simulink model "PIntkVUs_DD"  (R2016b)
settings: configuration reference "CodeGenConfigSet" (kept outside this file)
values from neighbouring files (symbols this model uses):
  Air_facPT1T1PIntkVUs_C = Calibration.Parameter    [init_PIntkVUs_DD.m]
  Air_pMaxDiffLimPlsPIntkVUs_C = Calibration.Parameter    [init_PIntkVUs_DD.m]
  Air_pMinDiffLimPlsPIntkVUs_C = Calibration.Parameter    [init_PIntkVUs_DD.m]
  Air_pPhysRngPIntkVUsMax_C = Calibration.Parameter    [init_PIntkVUs_DD.m]
  Air_pPhysRngPIntkVUsMin_C = Calibration.Parameter    [init_PIntkVUs_DD.m]
  Air_pTransfPIntkVUs_CUR = Calibration.Parameter    [init_PIntkVUs_DD.m]
  Air_pTransfPIntkVUs_CURX = Calibration.Parameter    [init_PIntkVUs_DD.m]
  Air_tiPhysRngHiIntkVUsDefDeb_C = Calibration.Parameter    [init_PIntkVUs_DD.m]
  Air_tiPhysRngHiIntkVUsOKDeb_C = Calibration.Parameter    [init_PIntkVUs_DD.m]
  Air_tiPhysRngLoIntkVUsDefDeb_C = Calibration.Parameter    [init_PIntkVUs_DD.m]
  Air_tiPhysRngLoIntkVUsOKDeb_C = Calibration.Parameter    [init_PIntkVUs_DD.m]
  Air_tiPIntkVUsMaxDefDeb_C = Calibration.Parameter    [init_PIntkVUs_DD.m]
  Air_tiPIntkVUsMaxOKDeb_C = Calibration.Parameter    [init_PIntkVUs_DD.m]
  Air_tiPIntkVUsMinDefDeb_C = Calibration.Parameter    [init_PIntkVUs_DD.m]
  Air_tiPIntkVUsMinOKDeb_C = Calibration.Parameter    [init_PIntkVUs_DD.m]
  Air_tiPlsMaxIntkVUsDefDeb_C = Calibration.Parameter    [init_PIntkVUs_DD.m]
  Air_tiPlsMaxIntkVUsOKDeb_C = Calibration.Parameter    [init_PIntkVUs_DD.m]
  Air_tiPlsMinIntkVUsDefDeb_C = Calibration.Parameter    [init_PIntkVUs_DD.m]
  Air_tiPlsMinIntkVUsOKDeb_C = Calibration.Parameter    [init_PIntkVUs_DD.m]
  Air_uSRCPIntkVUsMax_C = Calibration.Parameter    [init_PIntkVUs_DD.m]
  Air_uSRCPIntkVUsMin_C = Calibration.Parameter    [init_PIntkVUs_DD.m]
undefined symbols (not defined in the file or in its folder): EpmSynState_conv, PIntkVUs_DD_DT
libraries: CXLib x19
settings Model: Creator=GaberXu  LastModifiedBy=wangrui
settings ConfigSetRef: SourceLocation=Base Workspace

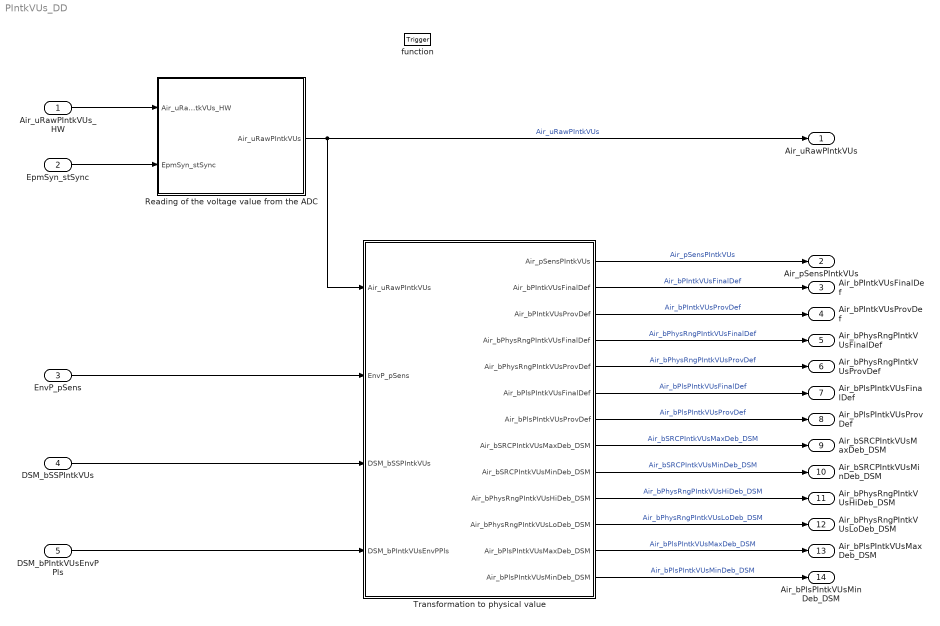
== system PIntkVUs_DD ==
  Air_uRawPIntkVUs_HW : Inport  Tag=mv  Description=Raw ADC value of air pressure upstream of the intake valve  OutMin=0  OutMax=5000  OutDataTypeStr=Ad_mv
  EpmSyn_stSync : Inport  Description=state of synchronization  Port=2  OutDataTypeStr=Enum:EpmSynState_conv
  EnvP_pSens : Inport  Tag=kPa  Description=Raw physical value  Port=3  OutMin=0  OutMax=1200  OutDataTypeStr=AirPressure_kPa
  DSM_bSSPIntkVUs : Inport  Description=State of FId_SSPIntkVUs  Port=4  OutMin=0  OutMax=1  OutDataTypeStr=boolean
  DSM_bPIntkVUsEnvPPls : Inport  Description=State of FId_PIntkVUsEnvPPls  Port=5  OutMin=0  OutMax=1  OutDataTypeStr=boolean
  function : TriggerPort  TriggerType=function-call  VariantControl=Variant
  Reading of the voltage value from the ADC : Subsystem
  Transformation to physical value : Subsystem
  Air_uRawPIntkVUs : Outport  Tag=mv  Description=Averaging raw ADC value of air pressure upstream of the intake valve  OutMin=0  OutMax=5000  OutDataTypeStr=Ad_mv
  Air_pSensPIntkVUs : Outport  Tag=kPa  Description=Sensed manifold absolute pressure  Port=2  OutMin=0  OutMax=1200  OutDataTypeStr=AirPressure_kPa
  Air_bPIntkVUsFinalDef : Outport  Description=Final defect of the raw air pressure upstream of the intake valve  Port=3  OutMin=0  OutMax=1  OutDataTypeStr=boolean
  Air_bPIntkVUsProvDef : Outport  Description=Provisional defect of the raw air pressure upstream of the intake valve  Port=4  OutMin=0  OutMax=1  OutDataTypeStr=boolean
  Air_bPhysRngPIntkVUsFinalDef : Outport  Description=Final defect of the physical air pressure upstream of the intake valve  Port=5  OutMin=0  OutMax=1  OutDataTypeStr=boolean
  Air_bPhysRngPIntkVUsProvDef : Outport  Description=Provisional defect of the physical air pressure upstream of the intake valve  Port=6  OutMin=0  OutMax=1  OutDataTypeStr=boolean
  Air_bPlsPIntkVUsFinalDef : Outport  Description=Final defect which the air pressure upstream of the intake valve is not plausible  Port=7  OutMin=0  OutMax=1  OutDataTypeStr=boolean
  Air_bPlsPIntkVUsProvDef : Outport  Description=Provisional defect which the air pressure upstream of the intake valve is not plausible  Port=8  OutMin=0  OutMax=1  OutDataTypeStr=boolean
  Air_bSRCPIntkVUsMaxDeb_DSM : Outport  Description=DSM defect which the raw air pressure upstream of the intake valve is exceeding the maximum in SRC  Port=9  OutMin=0  OutMax=1  OutDataTypeStr=boolean
  Air_bSRCPIntkVUsMinDeb_DSM : Outport  Description=DSM defect which the raw air pressure upstream of the intake valve is exceeding the minimum in SRC  Port=10  OutMin=0  OutMax=1  OutDataTypeStr=boolean
  Air_bPhysRngPIntkVUsHiDeb_DSM : Outport  Description="DSM defect which the physical  air pressure upstream of the intake valve is exceeding the highest value in SRC"  Port=11  OutMin=0  OutMax=1  OutDataTypeStr=boolean
  Air_bPhysRngPIntkVUsLoDeb_DSM : Outport  Description="DSM defect which the physical  air pressure upstream of the intake valve is exceeding the lowest value in SRC"  Port=12  OutMin=0  OutMax=1  OutDataTypeStr=boolean
  Air_bPlsPIntkVUsMaxDeb_DSM : Outport  Description=DSM defect which the air pressure upstream of the intake valve is exceeding the maximum in plausibility check  Port=13  OutMin=0  OutMax=1  OutDataTypeStr=boolean
  Air_bPlsPIntkVUsMinDeb_DSM : Outport  Description=DSM defect which the air pressure upstream of the intake valve is exceeding the minimum in plausibility check  Port=14  OutMin=0  OutMax=1  OutDataTypeStr=boolean
  wires:
  Reading of the voltage value from the ADC/1(Air_uRawPIntkVUs) -> Air_uRawPIntkVUs/1, Transformation to physical value/1(Air_uRawPIntkVUs)  "Air_uRawPIntkVUs"
  Transformation to physical value/1(Air_pSensPIntkVUs) -> Air_pSensPIntkVUs/1  "Air_pSensPIntkVUs"
  Transformation to physical value/2(Air_bPIntkVUsFinalDef) -> Air_bPIntkVUsFinalDef/1  "Air_bPIntkVUsFinalDef"
  Transformation to physical value/3(Air_bPIntkVUsProvDef) -> Air_bPIntkVUsProvDef/1  "Air_bPIntkVUsProvDef"
  Transformation to physical value/4(Air_bPhysRngPIntkVUsFinalDef) -> Air_bPhysRngPIntkVUsFinalDef/1  "Air_bPhysRngPIntkVUsFinalDef"
  Transformation to physical value/5(Air_bPhysRngPIntkVUsProvDef) -> Air_bPhysRngPIntkVUsProvDef/1  "Air_bPhysRngPIntkVUsProvDef"
  Transformation to physical value/6(Air_bPlsPIntkVUsFinalDef) -> Air_bPlsPIntkVUsFinalDef/1  "Air_bPlsPIntkVUsFinalDef"
  Transformation to physical value/7(Air_bPlsPIntkVUsProvDef) -> Air_bPlsPIntkVUsProvDef/1  "Air_bPlsPIntkVUsProvDef"
  Transformation to physical value/8(Air_bSRCPIntkVUsMaxDeb_DSM) -> Air_bSRCPIntkVUsMaxDeb_DSM/1  "Air_bSRCPIntkVUsMaxDeb_DSM"
  Transformation to physical value/9(Air_bSRCPIntkVUsMinDeb_DSM) -> Air_bSRCPIntkVUsMinDeb_DSM/1  "Air_bSRCPIntkVUsMinDeb_DSM"
  Transformation to physical value/10(Air_bPhysRngPIntkVUsHiDeb_DSM) -> Air_bPhysRngPIntkVUsHiDeb_DSM/1  "Air_bPhysRngPIntkVUsHiDeb_DSM"
  Transformation to physical value/11(Air_bPhysRngPIntkVUsLoDeb_DSM) -> Air_bPhysRngPIntkVUsLoDeb_DSM/1  "Air_bPhysRngPIntkVUsLoDeb_DSM"
  Transformation to physical value/12(Air_bPlsPIntkVUsMaxDeb_DSM) -> Air_bPlsPIntkVUsMaxDeb_DSM/1  "Air_bPlsPIntkVUsMaxDeb_DSM"
  Transformation to physical value/13(Air_bPlsPIntkVUsMinDeb_DSM) -> Air_bPlsPIntkVUsMinDeb_DSM/1  "Air_bPlsPIntkVUsMinDeb_DSM"
  EpmSyn_stSync/1 -> Reading of the voltage value from the ADC/2(EpmSyn_stSync)
  Air_uRawPIntkVUs_HW/1 -> Reading of the voltage value from the ADC/1(Air_uRawPIntkVUs_HW)
  EnvP_pSens/1 -> Transformation to physical value/2(EnvP_pSens)
  DSM_bSSPIntkVUs/1 -> Transformation to physical value/3(DSM_bSSPIntkVUs)
  DSM_bPIntkVUsEnvPPls/1 -> Transformation to physical value/4(DSM_bPIntkVUsEnvPPls)

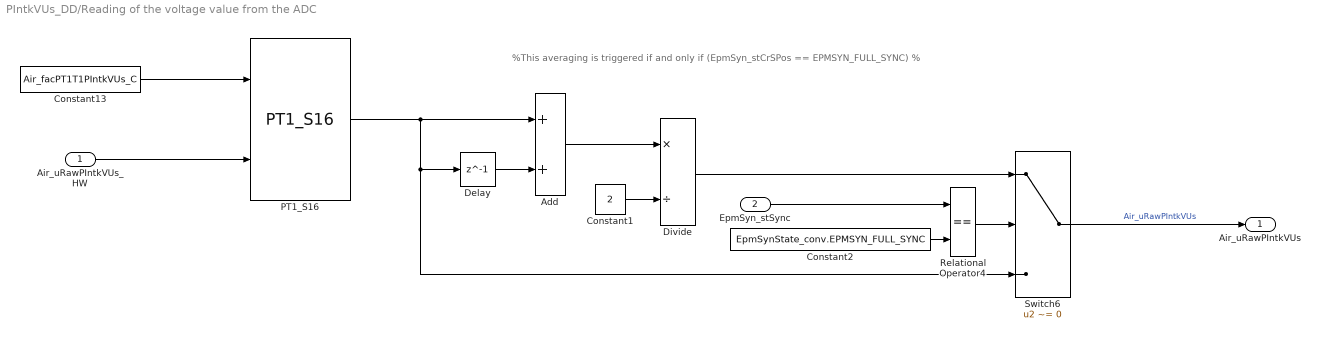
== system PIntkVUs_DD/Reading of the voltage value from the ADC ==
  note: %This averaging is triggered if and only if (EpmSyn_stCrSPos == EPMSYN_FULL_SYNC) %
  Air_uRawPIntkVUs_HW : Inport
  EpmSyn_stSync : Inport  Port=2
  Add : Sum  SaturateOnIntegerOverflow=on  InputSameDT=on
  Constant1 : Constant  Value=2  OutDataTypeStr=uint16
  Constant13 : Constant  Value=Air_facPT1T1PIntkVUs_C
  Constant2 : Constant  Value=EpmSynState_conv.EPMSYN_FULL_SYNC
  Delay : Delay  DelayLength=1  InitialCondition=0
  Divide : Product  Inputs=*/  OutDataTypeStr=Ad_mv  SaturateOnIntegerOverflow=on
  PT1_S16 : CXLib/PT1_S16  offset=0
  Relational Operator4 : RelationalOperator  Operator===  OutDataTypeStr=boolean  RndMeth=Nearest  InputSameDT=on
  Switch6 : Switch  Criteria=u2 ~= 0  InputSameDT=on
  Air_uRawPIntkVUs : Outport
  wires:
  Air_uRawPIntkVUs_HW/1 -> PT1_S16/2
  Constant1/1 -> Divide/2
  Relational Operator4/1 -> Switch6/2
  Divide/1 -> Switch6/1
  Delay/1 -> Add/2
  Switch6/1 -> Air_uRawPIntkVUs/1  "Air_uRawPIntkVUs"
  EpmSyn_stSync/1 -> Relational Operator4/1
  Add/1 -> Divide/1
  Constant2/1 -> Relational Operator4/2
  Constant13/1 -> PT1_S16/1
  PT1_S16/1 -> Switch6/3, Delay/1, Add/1

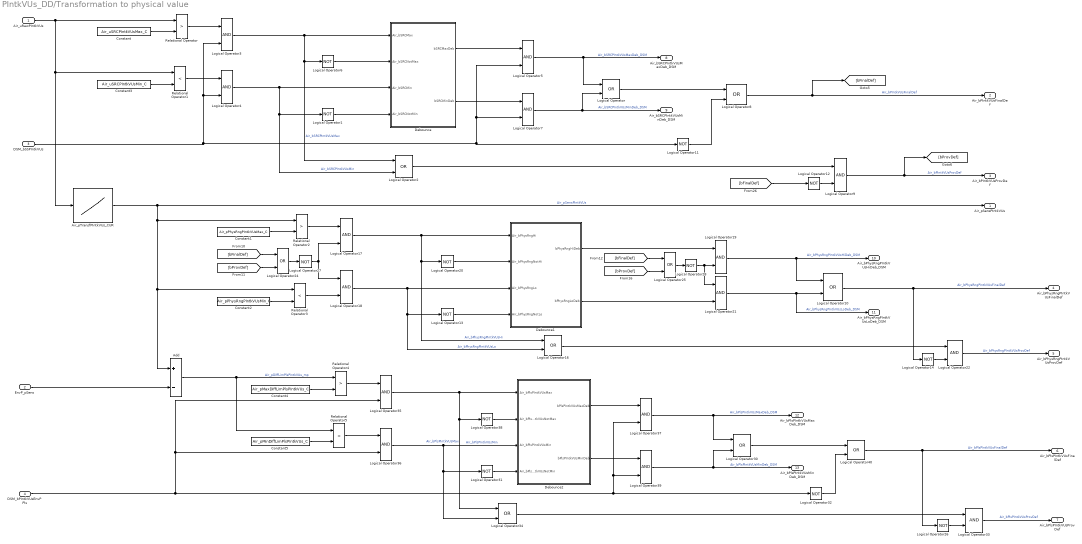
== system PIntkVUs_DD/Transformation to physical value ==
  Air_uRawPIntkVUs : Inport
  EnvP_pSens : Inport  Port=2
  DSM_bSSPIntkVUs : Inport  Port=3
  DSM_bPIntkVUsEnvPPls : Inport  Port=4
  Add : Sum  Inputs=+-  SaturateOnIntegerOverflow=on  InputSameDT=on
  Air_pTransfPIntkVUs_CUR : Lookup_n-D  NumberOfTableDimensions=1  BreakpointsForDimension1=Air_pTransfPIntkVUs_CURX  IndexSearchMethod=Linear search  BeginIndexSearchUsingPreviousIndexResult=on  UseOneInputPortForAllInputData=on  Table=Air_pTransfPIntkVUs_CUR  ExtrapMethod=Clip  UseLastTableValue=on  InternalRulePriority=Speed  OutDataTypeStr=Inherit: Inherit via back propagation  SaturateOnIntegerOverflow=on
  Constant : Constant  Value=Air_uSRCPIntkVUsMax_C
  Constant1 : Constant  Value=Air_pPhysRngPIntkVUsMax_C
  Constant2 : Constant  Value=Air_pPhysRngPIntkVUsMin_C
  Constant3 : Constant  Value=Air_uSRCPIntkVUsMin_C
  Constant4 : Constant  Value=Air_pMaxDiffLimPlsPIntkVUs_C
  Constant5 : Constant  Value=Air_pMinDiffLimPlsPIntkVUs_C
  Debounce : Subsystem
  Debounce1 : Subsystem
  Debounce2 : Subsystem
  Logical Operator{,2,8,10,16,30,34,40} (8 alike) : Logic  Operator=OR  AllPortsSameDT=off  OutDataTypeStr=boolean
  Logical Operator{1,6,11..14,20,26..28,31..32,38} (13 alike) : Logic  Operator=NOT  AllPortsSameDT=off  OutDataTypeStr=boolean
  Logical Operator{3..5,7,9,17..19,21..22,33,35..37,39} (15 alike) : Logic  AllPortsSameDT=off  OutDataTypeStr=boolean
  Logical Operator24 : Logic  RequirementInfo={} %GIDa_41b44013_9ec1_49ef_a77d_a735944319c0  Operator=OR  OutDataTypeStr=boolean
  Logical Operator25 : Logic  RequirementInfo={} %GIDa_cee60f6c_ce8d_407f_bb4c_290855d67459  Operator=OR  OutDataTypeStr=boolean
  Relational Operator : RelationalOperator  Operator=>  OutDataTypeStr=boolean  RndMeth=Nearest  InputSameDT=on
  Relational Operator1 : RelationalOperator  Operator=<  OutDataTypeStr=boolean  RndMeth=Nearest  InputSameDT=on
  Relational Operator2 : RelationalOperator  Operator=>  OutDataTypeStr=boolean  RndMeth=Nearest  InputSameDT=on
  Relational Operator3 : RelationalOperator  Operator=<  OutDataTypeStr=boolean  RndMeth=Nearest  InputSameDT=on
  Relational Operator4 : RelationalOperator  Operator=>  OutDataTypeStr=boolean  RndMeth=Nearest  InputSameDT=on
  Relational Operator5 : RelationalOperator  Operator=<  OutDataTypeStr=boolean  RndMeth=Nearest  InputSameDT=on
  Air_pSensPIntkVUs : Outport
  Air_bPIntkVUsFinalDef : Outport  Port=2
  Air_bPIntkVUsProvDef : Outport  Port=3
  Air_bPhysRngPIntkVUsFinalDef : Outport  Port=4
  Air_bPhysRngPIntkVUsProvDef : Outport  Port=5
  Air_bPlsPIntkVUsFinalDef : Outport  Port=6
  Air_bPlsPIntkVUsProvDef : Outport  Port=7
  Air_bSRCPIntkVUsMaxDeb_DSM : Outport  Port=8
  Air_bSRCPIntkVUsMinDeb_DSM : Outport  Port=9
  Air_bPhysRngPIntkVUsHiDeb_DSM : Outport  Port=10
  Air_bPhysRngPIntkVUsLoDeb_DSM : Outport  Port=11
  Air_bPlsPIntkVUsMaxDeb_DSM : Outport  Port=12
  Air_bPlsPIntkVUsMinDeb_DSM : Outport  Port=13
  wires:
  Logical Operator33/1 -> Air_bPlsPIntkVUsProvDef/1  "Air_bPlsPIntkVUsProvDef"
  Logical Operator34/1 -> Logical Operator33/1
  Logical Operator26/1 -> Logical Operator33/2
  Logical Operator22/1 -> Air_bPhysRngPIntkVUsProvDef/1  "Air_bPhysRngPIntkVUsProvDef"
  Logical Operator14/1 -> Logical Operator22/2
  Debounce2/1(bPlsPIntkVUsMaxDeb) -> Logical Operator37/1
  Logical Operator31/1 -> Debounce2/4(Air_bPlsPIntkVUsNotMin)
  Logical Operator38/1 -> Debounce2/2(Air_bPlsPIntkVUsNotMax)
  Add/1 -> Relational Operator4/1, Relational Operator5/1  "Air_pDiffLimPlsPIntkVUs_mp"
  Logical Operator32/1 -> Logical Operator40/2
  Logical Operator40/1 -> Air_bPlsPIntkVUsFinalDef/1, Logical Operator26/1  "Air_bPlsPIntkVUsFinalDef"
  DSM_bPIntkVUsEnvPPls/1 -> Logical Operator32/1, Logical Operator37/2, Logical Operator39/2, Logical Operator35/2, Logical Operator36/2
  Logical Operator30/1 -> Logical Operator40/1
  Debounce2/2(bPlsPIntkVUsMinDeb) -> Logical Operator39/1
  Relational Operator5/1 -> Logical Operator36/1
  Relational Operator4/1 -> Logical Operator35/1
  Logical Operator39/1 -> Logical Operator30/2, Air_bPlsPIntkVUsMinDeb_DSM/1  "Air_bPlsPIntkVUsMinDeb_DSM"
  Logical Operator37/1 -> Air_bPlsPIntkVUsMaxDeb_DSM/1, Logical Operator30/1  "Air_bPlsPIntkVUsMaxDeb_DSM"
  Logical Operator36/1 -> Debounce2/3(Air_bPlsPIntkVUsMin), Logical Operator34/2, Logical Operator31/1  "Air_bPlsPIntkVUsMin"
  Constant5/1 -> Relational Operator5/2
  Logical Operator35/1 -> Debounce2/1(Air_bPlsPIntkVUsMax), Logical Operator34/1, Logical Operator38/1  "Air_bPlsPIntkVUsMax"
  Constant4/1 -> Relational Operator4/2
  EnvP_pSens/1 -> Add/2
  Logical Operator28/1 -> Logical Operator19/2, Logical Operator21/1
  Logical Operator27/1 -> Logical Operator17/2, Logical Operator18/1
  Debounce1/2(bPhysRngLoDeb) -> Logical Operator21/2
  [bProvDef] -> Logical Operator25/2
  [bFinalDef] -> Logical Operator25/1
  [bProvDef] -> Logical Operator24/2
  [bFinalDef] -> Logical Operator24/1
  Relational Operator3/1 -> Logical Operator18/2
  Debounce1/1(bPhysRngHiDeb) -> Logical Operator19/1
  Logical Operator13/1 -> Debounce1/4(Air_bPhysRngNotLo)
  Logical Operator20/1 -> Debounce1/2(Air_bPhysRngNotHi)
  Logical Operator10/1 -> Logical Operator14/1, Air_bPhysRngPIntkVUsFinalDef/1  "Air_bPhysRngPIntkVUsFinalDef"
  Logical Operator16/1 -> Logical Operator22/1
  Logical Operator25/1 -> Logical Operator28/1
  Logical Operator24/1 -> Logical Operator27/1
  Relational Operator2/1 -> Logical Operator17/1
  Logical Operator21/1 -> Air_bPhysRngPIntkVUsLoDeb_DSM/1, Logical Operator10/2  "Air_bPhysRngPIntkVUsLoDeb_DSM"
  Logical Operator19/1 -> Air_bPhysRngPIntkVUsHiDeb_DSM/1, Logical Operator10/1  "Air_bPhysRngPIntkVUsHiDeb_DSM"
  Logical Operator18/1 -> Debounce1/3(Air_bPhysRngLo), Logical Operator16/2, Logical Operator13/1  "Air_bPhysRngPIntkVUsLo"
  Constant2/1 -> Relational Operator3/2
  Logical Operator17/1 -> Debounce1/1(Air_bPhysRngHi), Logical Operator20/1, Logical Operator16/1  "Air_bPhysRngPIntkVUsHi"
  Constant1/1 -> Relational Operator2/2
  Air_pTransfPIntkVUs_CUR/1 -> Relational Operator2/1, Relational Operator3/1, Add/1, Air_pSensPIntkVUs/1  "Air_pSensPIntkVUs"
  Debounce/2(bSRCMinDeb) -> Logical Operator7/1
  Debounce/1(bSRCMaxDeb) -> Logical Operator5/1
  Logical Operator1/1 -> Debounce/4(Air_bSRCNotMin)
  Logical Operator6/1 -> Debounce/2(Air_bSRCNotMax)
  Air_uRawPIntkVUs/1 -> Relational Operator/1, Relational Operator1/1, Air_pTransfPIntkVUs_CUR/1
  Logical Operator12/1 -> Logical Operator9/2
  Logical Operator11/1 -> Logical Operator8/2
  Logical Operator9/1 -> [bProvDef], Air_bPIntkVUsProvDef/1  "Air_bPIntkVUsProvDef"
  Logical Operator8/1 -> Air_bPIntkVUsFinalDef/1, [bFinalDef]  "Air_bPIntkVUsFinalDef"
  [bFinalDef] -> Logical Operator12/1
  Logical Operator2/1 -> Logical Operator9/1
  DSM_bSSPIntkVUs/1 -> Logical Operator5/2, Logical Operator7/2, Logical Operator11/1, Logical Operator3/2, Logical Operator4/2
  Logical Operator/1 -> Logical Operator8/1
  Relational Operator1/1 -> Logical Operator4/1
  Relational Operator/1 -> Logical Operator3/1
  Logical Operator7/1 -> Air_bSRCPIntkVUsMinDeb_DSM/1, Logical Operator/2  "Air_bSRCPIntkVUsMinDeb_DSM"
  Logical Operator5/1 -> Air_bSRCPIntkVUsMaxDeb_DSM/1, Logical Operator/1  "Air_bSRCPIntkVUsMaxDeb_DSM"
  Logical Operator4/1 -> Debounce/3(Air_bSRCMin), Logical Operator1/1, Logical Operator2/2  "Air_bSRCPIntkVUsMin"
  Constant3/1 -> Relational Operator1/2
  Logical Operator3/1 -> Debounce/1(Air_bSRCMax), Logical Operator6/1, Logical Operator2/1  "Air_bSRCPIntkVUsMax"
  Constant/1 -> Relational Operator/2

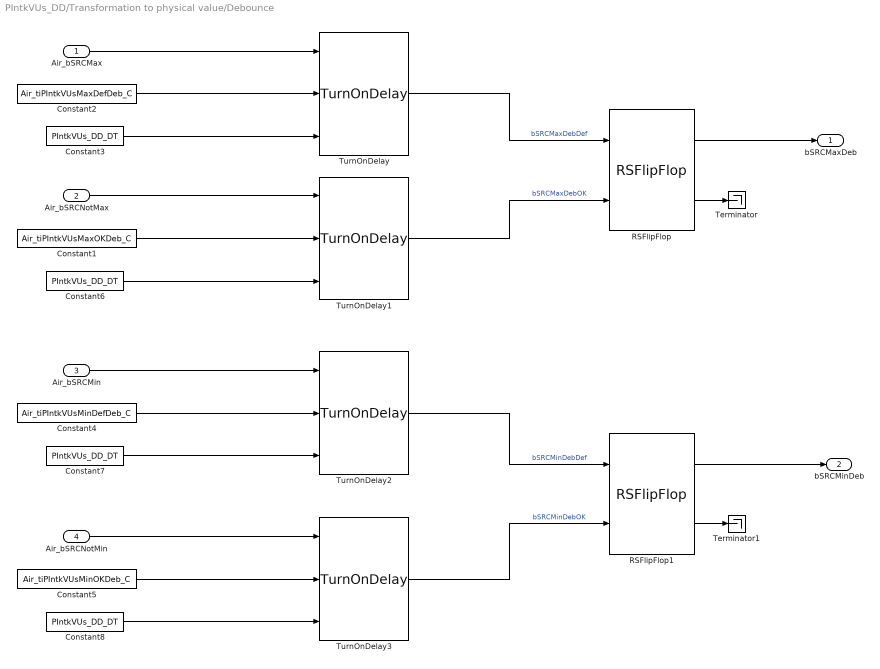
== system PIntkVUs_DD/Transformation to physical value/Debounce ==
  Air_bSRCMax : Inport
  Air_bSRCNotMax : Inport  Port=2
  Air_bSRCMin : Inport  Port=3
  Air_bSRCNotMin : Inport  Port=4
  Constant1 : Constant  Value=Air_tiPIntkVUsMaxOKDeb_C
  Constant2 : Constant  Value=Air_tiPIntkVUsMaxDefDeb_C
  Constant{3,6..8} (4 alike) : Constant  Value=PIntkVUs_DD_DT
  Constant4 : Constant  Value=Air_tiPIntkVUsMinDefDeb_C
  Constant5 : Constant  Value=Air_tiPIntkVUsMinOKDeb_C
  RSFlipFlop : CXLib/RSFlipFlop
  RSFlipFlop1 : CXLib/RSFlipFlop
  Terminator : Terminator
  Terminator1 : Terminator
  TurnOnDelay{,1..3} (4 alike) : CXLib/TurnOnDelay
  bSRCMaxDeb : Outport
  bSRCMinDeb : Outport  Port=2
  wires:
  Constant8/1 -> TurnOnDelay3/3
  Constant7/1 -> TurnOnDelay2/3
  Constant6/1 -> TurnOnDelay1/3
  Constant3/1 -> TurnOnDelay/3
  Air_bSRCMax/1 -> TurnOnDelay/1
  RSFlipFlop1/2 -> Terminator1/1
  RSFlipFlop/2 -> Terminator/1
  Constant5/1 -> TurnOnDelay3/2
  TurnOnDelay3/1 -> RSFlipFlop1/2  "bSRCMinDebOK"
  Air_bSRCNotMin/1 -> TurnOnDelay3/1
  TurnOnDelay2/1 -> RSFlipFlop1/1  "bSRCMinDebDef"
  Air_bSRCMin/1 -> TurnOnDelay2/1
  Air_bSRCNotMax/1 -> TurnOnDelay1/1
  TurnOnDelay/1 -> RSFlipFlop/1  "bSRCMaxDebDef"
  Constant2/1 -> TurnOnDelay/2
  Constant1/1 -> TurnOnDelay1/2
  Constant4/1 -> TurnOnDelay2/2
  TurnOnDelay1/1 -> RSFlipFlop/2  "bSRCMaxDebOK"
  RSFlipFlop/1 -> bSRCMaxDeb/1
  RSFlipFlop1/1 -> bSRCMinDeb/1

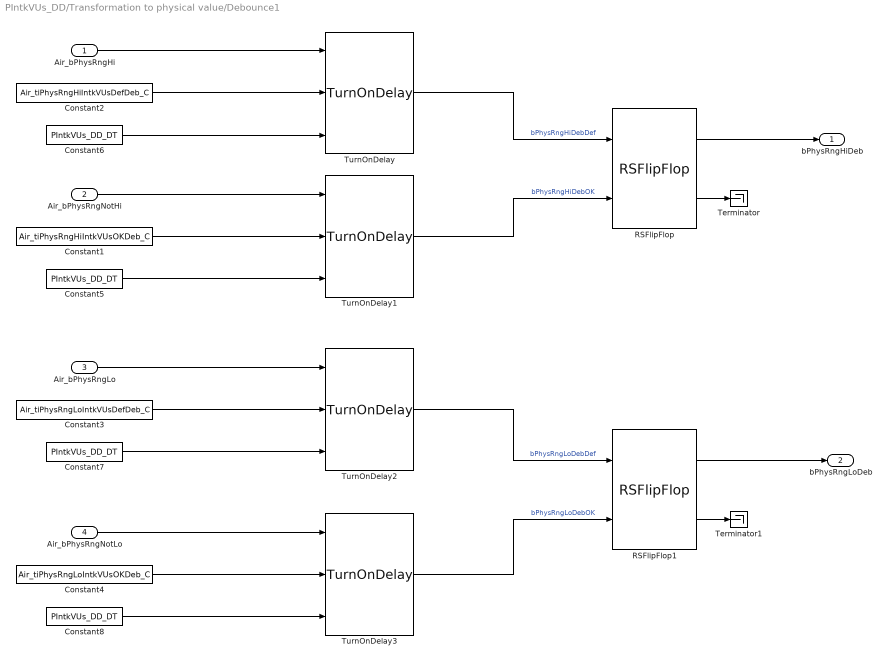
== system PIntkVUs_DD/Transformation to physical value/Debounce1 ==
  Air_bPhysRngHi : Inport
  Air_bPhysRngNotHi : Inport  Port=2
  Air_bPhysRngLo : Inport  Port=3
  Air_bPhysRngNotLo : Inport  Port=4
  Constant1 : Constant  Value=Air_tiPhysRngHiIntkVUsOKDeb_C
  Constant2 : Constant  Value=Air_tiPhysRngHiIntkVUsDefDeb_C
  Constant3 : Constant  Value=Air_tiPhysRngLoIntkVUsDefDeb_C
  Constant4 : Constant  Value=Air_tiPhysRngLoIntkVUsOKDeb_C
  Constant{5..8} (4 alike) : Constant  Value=PIntkVUs_DD_DT
  RSFlipFlop : CXLib/RSFlipFlop
  RSFlipFlop1 : CXLib/RSFlipFlop
  Terminator : Terminator
  Terminator1 : Terminator
  TurnOnDelay{,1..3} (4 alike) : CXLib/TurnOnDelay
  bPhysRngHiDeb : Outport
  bPhysRngLoDeb : Outport  Port=2
  wires:
  Constant8/1 -> TurnOnDelay3/3
  Constant7/1 -> TurnOnDelay2/3
  Constant5/1 -> TurnOnDelay1/3
  Constant6/1 -> TurnOnDelay/3
  RSFlipFlop1/1 -> bPhysRngLoDeb/1
  RSFlipFlop/1 -> bPhysRngHiDeb/1
  TurnOnDelay1/1 -> RSFlipFlop/2  "bPhysRngHiDebOK"
  Constant3/1 -> TurnOnDelay2/2
  Constant1/1 -> TurnOnDelay1/2
  Constant2/1 -> TurnOnDelay/2
  TurnOnDelay/1 -> RSFlipFlop/1  "bPhysRngHiDebDef"
  Air_bPhysRngNotHi/1 -> TurnOnDelay1/1
  Air_bPhysRngLo/1 -> TurnOnDelay2/1
  TurnOnDelay2/1 -> RSFlipFlop1/1  "bPhysRngLoDebDef"
  Air_bPhysRngNotLo/1 -> TurnOnDelay3/1
  TurnOnDelay3/1 -> RSFlipFlop1/2  "bPhysRngLoDebOK"
  Constant4/1 -> TurnOnDelay3/2
  RSFlipFlop/2 -> Terminator/1
  RSFlipFlop1/2 -> Terminator1/1
  Air_bPhysRngHi/1 -> TurnOnDelay/1

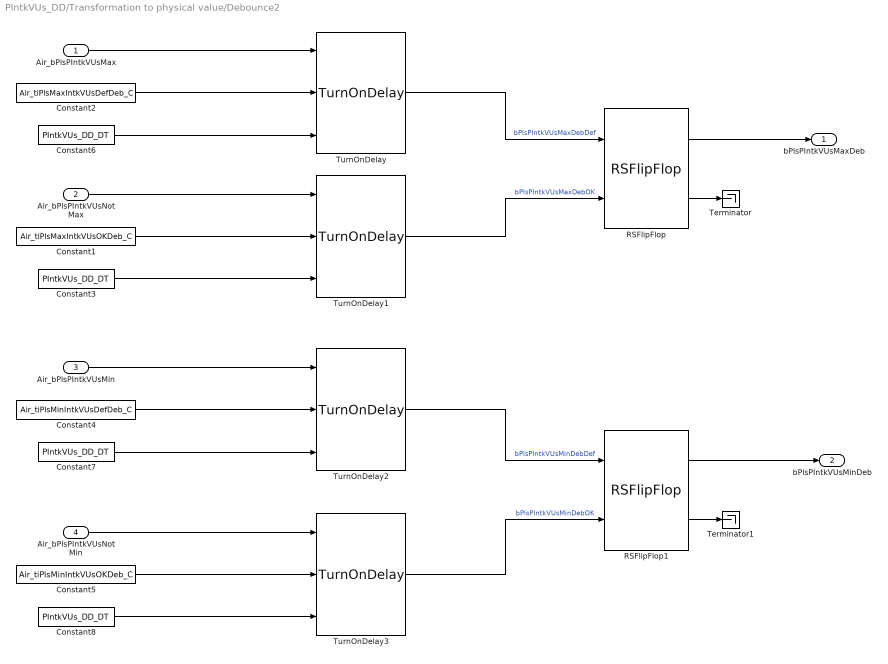
== system PIntkVUs_DD/Transformation to physical value/Debounce2 ==
  Air_bPlsPIntkVUsMax : Inport
  Air_bPlsPIntkVUsNotMax : Inport  Port=2
  Air_bPlsPIntkVUsMin : Inport  Port=3
  Air_bPlsPIntkVUsNotMin : Inport  Port=4
  Constant1 : Constant  Value=Air_tiPlsMaxIntkVUsOKDeb_C
  Constant2 : Constant  Value=Air_tiPlsMaxIntkVUsDefDeb_C
  Constant{3,6..8} (4 alike) : Constant  Value=PIntkVUs_DD_DT
  Constant4 : Constant  Value=Air_tiPlsMinIntkVUsDefDeb_C
  Constant5 : Constant  Value=Air_tiPlsMinIntkVUsOKDeb_C
  RSFlipFlop : CXLib/RSFlipFlop
  RSFlipFlop1 : CXLib/RSFlipFlop
  Terminator : Terminator
  Terminator1 : Terminator
  TurnOnDelay{,1..3} (4 alike) : CXLib/TurnOnDelay
  bPlsPIntkVUsMaxDeb : Outport
  bPlsPIntkVUsMinDeb : Outport  Port=2
  wires:
  Constant8/1 -> TurnOnDelay3/3
  Constant7/1 -> TurnOnDelay2/3
  Constant3/1 -> TurnOnDelay1/3
  Constant6/1 -> TurnOnDelay/3
  RSFlipFlop1/1 -> bPlsPIntkVUsMinDeb/1
  RSFlipFlop/1 -> bPlsPIntkVUsMaxDeb/1
  TurnOnDelay1/1 -> RSFlipFlop/2  "bPlsPIntkVUsMaxDebOK"
  Constant4/1 -> TurnOnDelay2/2
  Constant1/1 -> TurnOnDelay1/2
  Constant2/1 -> TurnOnDelay/2
  TurnOnDelay/1 -> RSFlipFlop/1  "bPlsPIntkVUsMaxDebDef"
  Air_bPlsPIntkVUsNotMax/1 -> TurnOnDelay1/1
  Air_bPlsPIntkVUsMin/1 -> TurnOnDelay2/1
  TurnOnDelay2/1 -> RSFlipFlop1/1  "bPlsPIntkVUsMinDebDef"
  Air_bPlsPIntkVUsNotMin/1 -> TurnOnDelay3/1
  TurnOnDelay3/1 -> RSFlipFlop1/2  "bPlsPIntkVUsMinDebOK"
  Constant5/1 -> TurnOnDelay3/2
  RSFlipFlop/2 -> Terminator/1
  RSFlipFlop1/2 -> Terminator1/1
  Air_bPlsPIntkVUsMax/1 -> TurnOnDelay/1
